simulink model "batteryMine"  (R2019a)
settings: Solver=ode4  StartTime=0.0  StopTime=125  FixedStep=.01  RelTol=1e-3
InitFcn:
  | addpath fcns;
  | load newBattery.mat;
libraries: simulink x2
settings Model: Creator=tdarrah  LastModifiedBy=tdarrah
settings DebuggingCC: ArithmeticOperatorsInVariantConditions=warning

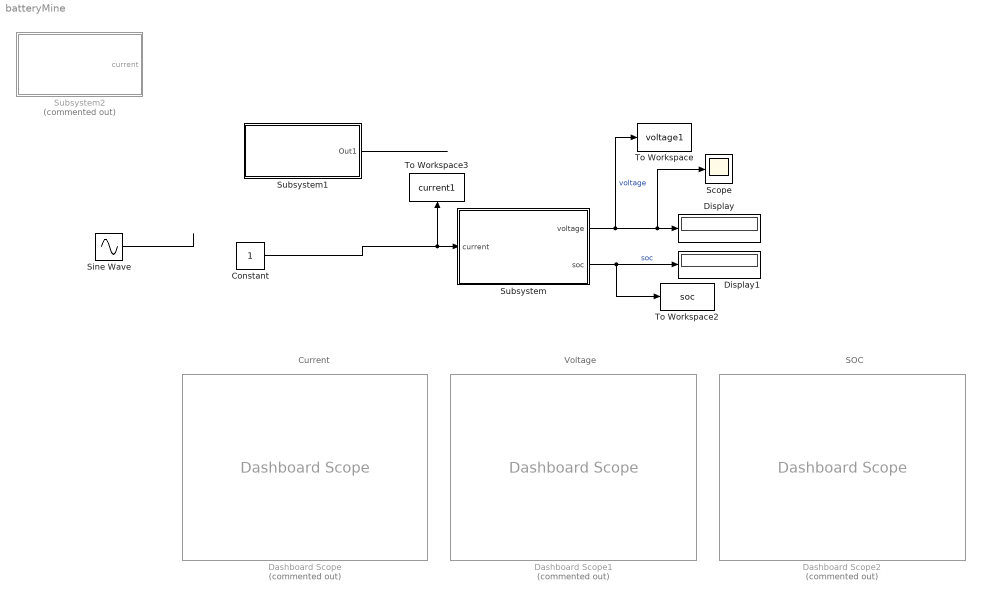
== system batteryMine ==
  note: Current
  note: Voltage
  note: SOC
  Constant : Constant
  Dashboard Scope : DashboardScope  Commented=on  Ymin=-5  Ymax=10
  Dashboard Scope1 : DashboardScope  Commented=on  Ymin=8  Ymax=13
  Dashboard Scope2 : DashboardScope  Commented=on
  Display : Display
  Display1 : Display
  Scope : Scope
  Sine Wave : Sin  SampleTime=0
  Subsystem : Subsystem
  Subsystem1 : Subsystem
  Subsystem2 : Subsystem  Commented=on
  To Workspace : ToWorkspace  VariableName=voltage1  SaveFormat=Timeseries  SampleTime=-1
  To Workspace2 : ToWorkspace  VariableName=soc  SaveFormat=Timeseries  SampleTime=-1
  To Workspace3 : ToWorkspace  VariableName=current1  SaveFormat=Timeseries  SampleTime=-1
  wires:
  Subsystem/1(voltage) -> To Workspace/1, Scope/1, Display/1  "voltage"
  Subsystem/2(soc) -> To Workspace2/1, Display1/1  "soc"
  Subsystem1/1(Out1) -> ?
  Sine Wave/1 -> ?
  Constant/1 -> To Workspace3/1, Subsystem/1(current)

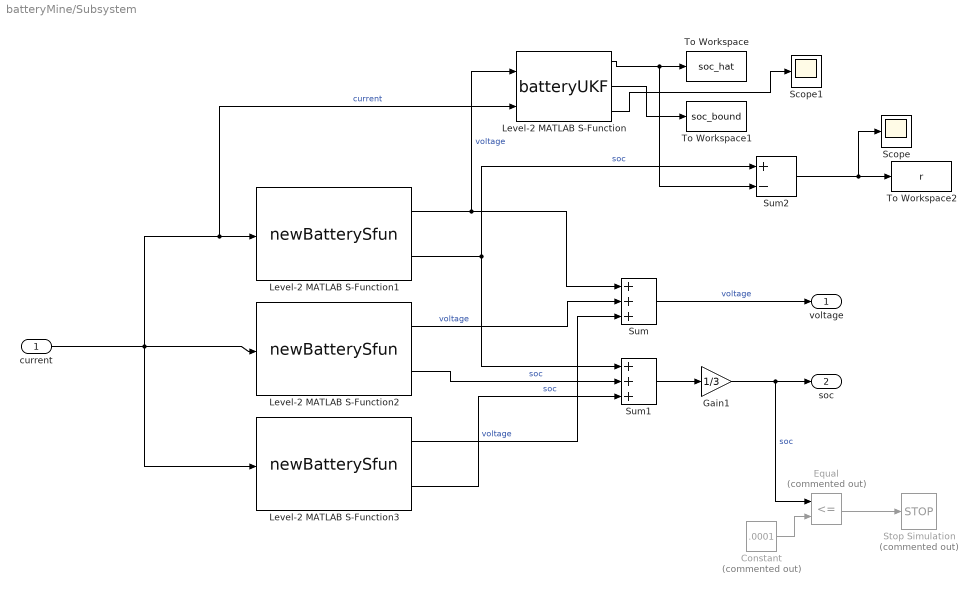
== system batteryMine/Subsystem ==
  current : Inport
  Constant : Constant  Commented=on  Value=.0001
  Equal : RelationalOperator  Commented=on  Operator=<=  OutDataTypeStr=boolean  RndMeth=Simplest
  Gain1 : Gain  Gain=1/3
  Level-2 MATLAB S-Function : M-S-Function  FunctionName=batteryUKF  Parameters=battery, .01, params
  Level-2 MATLAB S-Function1 : M-S-Function  FunctionName=newBatterySfun  Parameters=battery, .01
      mask Display:
      | port_label('input', 1, 'current');
      | port_label('output', 1, 'voltage');
      | port_label('output', 2, 'soc');
      | 
      | disp("Battery Cell");
  Level-2 MATLAB S-Function2 : M-S-Function  FunctionName=newBatterySfun  Parameters=battery, .01
      mask Display:
      | port_label('input', 1, 'current');
      | port_label('output', 1, 'voltage');
      | port_label('output', 2, 'soc');
  Level-2 MATLAB S-Function3 : M-S-Function  FunctionName=newBatterySfun  Parameters=battery, .01
      mask Display:
      | port_label('input', 1, 'current');
      | port_label('output', 1, 'voltage');
      | port_label('output', 2, 'soc');
  Scope : Scope
  Scope1 : Scope
  Stop Simulation : Stop  Commented=on
  Sum : Sum  Inputs=+++
  Sum1 : Sum  Inputs=+++
  Sum2 : Sum  Inputs=+-
  To Workspace : ToWorkspace  VariableName=soc_hat  SaveFormat=Timeseries  SampleTime=-1
  To Workspace1 : ToWorkspace  VariableName=soc_bound  SaveFormat=Timeseries  SampleTime=-1
  To Workspace2 : ToWorkspace  VariableName=r  SaveFormat=Timeseries  SampleTime=-1
  voltage : Outport
  soc : Outport  Port=2
  wires:
  Level-2 MATLAB S-Function2/1 -> Sum/2  "voltage"
  Level-2 MATLAB S-Function1/1 -> Level-2 MATLAB S-Function/1, Sum/1  "voltage"
  Level-2 MATLAB S-Function2/2 -> Sum1/2  "soc"
  Sum1/1 -> Gain1/1
  Gain1/1 -> Equal/1, soc/1  "soc"
  Level-2 MATLAB S-Function1/2 -> Sum2/1, Sum1/1  "soc"
  Level-2 MATLAB S-Function3/2 -> Sum1/3  "soc"
  current/1 -> Level-2 MATLAB S-Function3/1, Level-2 MATLAB S-Function/2, Level-2 MATLAB S-Function1/1, Level-2 MATLAB S-Function2/1  "current"
  Level-2 MATLAB S-Function3/1 -> Sum/3  "voltage"
  Sum/1 -> voltage/1  "voltage"
  Constant/1 -> Equal/2
  Equal/1 -> Stop Simulation/1
  Level-2 MATLAB S-Function/1 -> Sum2/2, To Workspace/1
  Level-2 MATLAB S-Function/2 -> To Workspace1/1
  Sum2/1 -> Scope/1, To Workspace2/1
  Level-2 MATLAB S-Function/3 -> Scope1/1

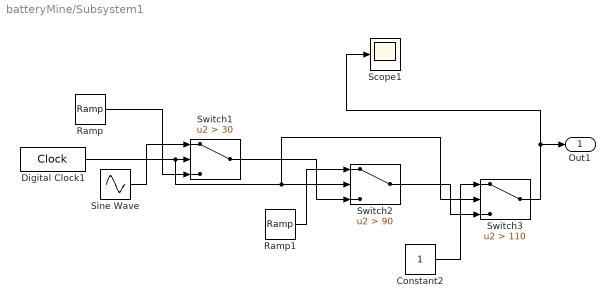
== system batteryMine/Subsystem1 ==
  Constant2 : Constant
  Digital Clock1 : DigitalClock
  Ramp : simulink/Sources/Ramp  slope=.025  start=1  InitialOutput=0
  Ramp1 : simulink/Sources/Ramp  slope=.05  start=90  InitialOutput=0
  Scope1 : Scope
  Sine Wave : Sin  SampleTime=0
  Switch1 : Switch  Criteria=u2 > Threshold  Threshold=30
  Switch2 : Switch  Criteria=u2 > Threshold  Threshold=90
  Switch3 : Switch  Criteria=u2 > Threshold  Threshold=110
  Out1 : Outport
  wires:
  Ramp1/1 -> Switch2/1
  Constant2/1 -> Switch3/1
  Ramp/1 -> Switch1/3
  Digital Clock1/1 -> Switch3/2, Switch2/2, Switch1/2
  Switch1/1 -> Switch2/3
  Sine Wave/1 -> Switch1/1
  Switch3/1 -> Out1/1, Scope1/1
  Switch2/1 -> Switch3/3

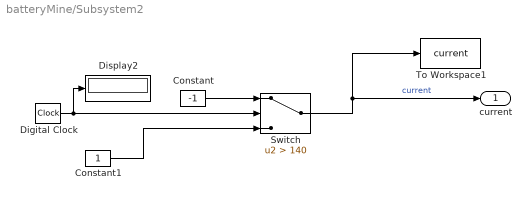
== system batteryMine/Subsystem2 ==
  Constant : Constant  Value=-1
  Constant1 : Constant
  Digital Clock : DigitalClock
  Display2 : Display
  Switch : Switch  Criteria=u2 > Threshold  Threshold=140
  To Workspace1 : ToWorkspace  VariableName=current  SaveFormat=Timeseries  SampleTime=.01
  current : Outport
  wires:
  Constant/1 -> Switch/1
  Switch/1 -> current/1, To Workspace1/1  "current"
  Digital Clock/1 -> Display2/1, Switch/2
  Constant1/1 -> Switch/3
